simulink model "lego_code"  (R2018a)
settings: Solver=FixedStepDiscrete  StartTime=0.0  StopTime=Tsim  FixedStep=Ts  RelTol=1e-3
InitFcn:
  | singleinvertedpendulum
values from neighbouring files (symbols this model uses):
  K2 = -K2    [singleinvertedpendulum.m]
  R = 0.021    [singleinvertedpendulum.m]
  Ts = 0.001    [singleinvertedpendulum.m]
  x0 = [0;0.1;0;0]    [singleinvertedpendulum.m]
undefined symbols (not defined in the file or in its folder): Ad, Bd, Cd, Dd, Discrete, Time
libraries: legoev3lib x5, ctrlSharedLib x1
settings Model: ExtModeTrigDuration=2  Creator=srivats  LastModifiedBy=srivats
settings SolverCC: PositivePriorityOrder=on
settings OptimizationCC: EnhancedBackFolding=on  PassReuseOutputArgsAs=Individual arguments  MaxStackSize=64  OptimizeBlockOrder=speed  DifferentSizesBufferReuse=on  OptimizationCustomize=off
settings DebuggingCC: ParameterTunabilityLossMsg=error
settings HardwareCC: ProdBitPerPointer=32  ProdBitPerSizeT=32  ProdBitPerPtrDiffT=32  ProdLargestAtomicInteger=Long  ProdWordSize=32  ProdHWDeviceType=ARM Compatible->ARM 9
settings SFSimCC: MATLABDynamicMemAlloc=off
settings RTWCC: SystemTargetFile=ert.tlc  HardwareBoard=LEGO MINDSTORMS EV3  TLCOptions="-aInlineSetEventsForThisBaseRateFcn=TLC_FALSE -aSuppressMultiTaskScheduler=TLC_FALSE  -aRateBasedStepFcn=0"  TemplateMakefile=ert_default_tmf  GenerateReport=on  Toolchain=Sourcery G++ Lite v2009q3  IncludeHyperlinkInReport=on  LaunchReport=on  GenerateTraceInfo=on  GenerateTraceReport=on  GenerateTraceReportSl=on  GenerateTraceReportSf=on  GenerateTraceReportEml=on
settings CodeAppCC: ForceParamTrailComments=on  IgnoreCustomStorageClasses=off  OperatorAnnotations=on  SimulinkDataObjDesc=on  SFDataObjDesc=on  InsertBlockDesc=on
settings ERTTargetCC: SupportContinuousTime=on  SupportVariableSizeSignals=on

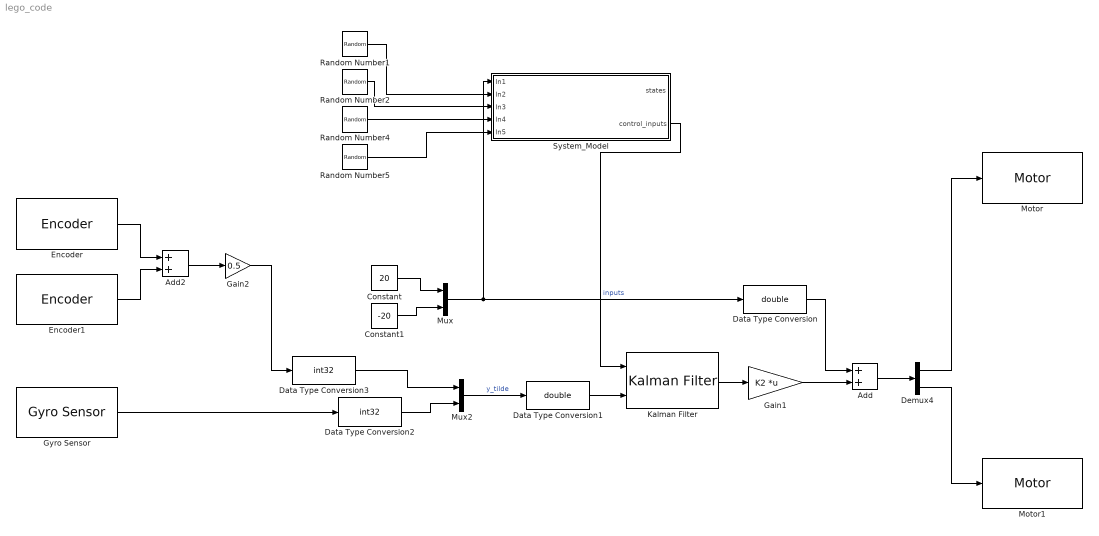
== system lego_code ==
  Add : Sum
  Add2 : Sum
  Constant : Constant  Value=20
  Constant1 : Constant  Value=-20
  Data Type Conversion : DataTypeConversion  OutDataTypeStr=double
  Data Type Conversion1 : DataTypeConversion  OutDataTypeStr=double
  Data Type Conversion2 : DataTypeConversion  OutDataTypeStr=int32
  Data Type Conversion3 : DataTypeConversion  OutDataTypeStr=int32
  Demux4 : Demux  Outputs=2
  Encoder : legoev3lib/Encoder  portNumber=A  opMode=Reset at each sample time  sampleTime=Ts
      settings: SourceProductName=Simulink Support Package for LEGO MINDSTORMS EV3 Hardware  SourceProductBaseCode=LEGOEV3
  Encoder1 : legoev3lib/Encoder  portNumber=D  opMode=Reset at each sample time  sampleTime=Ts
      settings: SourceProductName=Simulink Support Package for LEGO MINDSTORMS EV3 Hardware  SourceProductBaseCode=LEGOEV3
  Gain1 : Gain  Gain=K2  Multiplication=Matrix(K*u)
  Gain2 : Gain  Gain=0.5
  Gyro Sensor : legoev3lib/Gyro Sensor  portNumber=2  sampleTime=Ts
      settings: SourceProductName=Simulink Support Package for LEGO MINDSTORMS EV3 Hardware  SourceProductBaseCode=LEGOEV3
  Kalman Filter : ctrlSharedLib/Kalman Filter  TimeDomain=Discrete-Time  UseCurrentEstimator=on  ModelSource=Individual A, B, C, D matrices  ModelSourceVariable=ss(0.95,1,1,0,1)  A=Ad  B=Bd  C=Cd  D=Dd  NumberOfStates=4  NumberOfInputs=2  NumberOfOutputs=2  InitialEstimateSource=Dialog  X0=x0  P0=P0  UseK=off  UseGH=off  NumberOfProcessNoiseInputs=1  G=1  TimeInvariantG=on  H=0  TimeInvariantH=on  Q=Q  TimeInvariantQ=on  R=R  TimeInvariantR=on  N=0  TimeInvariantN=on  AddInputPort=on  AddEnablePort=off  OutputEstimatedY=off  OutputP=off  Ts=-1
      settings: SourceProductBaseCode=CT
  Motor : legoev3lib/Motor  sportNumber=A  sstopAction=Brake
  Motor1 : legoev3lib/Motor  sportNumber=D  sstopAction=Brake
  Mux : Mux  Inputs=2
  Mux2 : Mux  Inputs=2
  Random Number1 : RandomNumber  Variance=0.01  SampleTime=Ts
  Random Number2 : RandomNumber  Variance=0.025  Seed=1  SampleTime=Ts
  Random Number4 : RandomNumber  Variance=0.025  Seed=1  SampleTime=Ts
  Random Number5 : RandomNumber  Variance=0.025  Seed=1  SampleTime=Ts
  System_Model : Subsystem
  wires:
  Add/1 -> Demux4/1
  Kalman Filter/1 -> Gain1/1
  Demux4/1 -> Motor/1
  Gain1/1 -> Add/2
  Demux4/2 -> Motor1/1
  Data Type Conversion/1 -> Add/1
  Data Type Conversion1/1 -> Kalman Filter/2
  Constant1/1 -> Mux/2
  Constant/1 -> Mux/1
  Random Number2/1 -> System_Model/3(In3)
  Random Number5/1 -> System_Model/5(In5)
  Mux/1 -> System_Model/1(In1), Data Type Conversion/1  "inputs"
  Random Number1/1 -> System_Model/2(In2)
  Random Number4/1 -> System_Model/4(In4)
  System_Model/2(control_inputs) -> Kalman Filter/1
  Data Type Conversion3/1 -> Mux2/1
  Data Type Conversion2/1 -> Mux2/2
  Gain2/1 -> Data Type Conversion3/1
  Encoder1/1 -> Add2/2
  Gyro Sensor/1 -> Data Type Conversion2/1
  Mux2/1 -> Data Type Conversion1/1  "y_tilde"
  Add2/1 -> Gain2/1
  Encoder/1 -> Add2/1

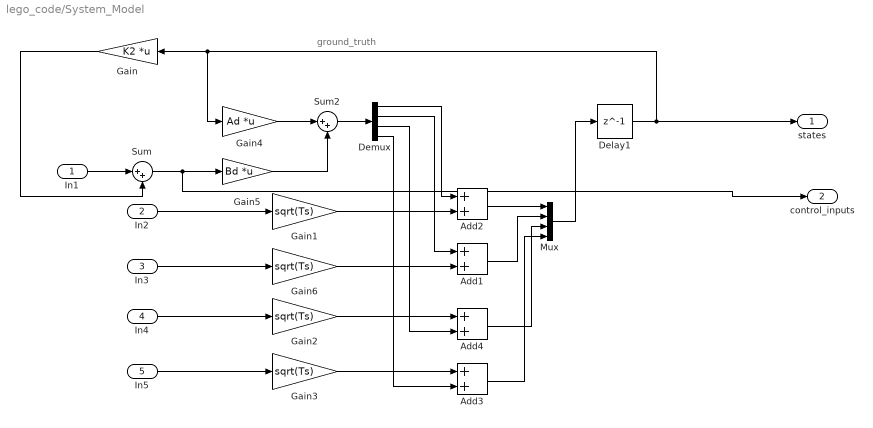
== system lego_code/System_Model ==
  note: ground_truth
  In1 : Inport
  In2 : Inport  Port=2
  In3 : Inport  Port=3
  In4 : Inport  Port=4
  In5 : Inport  Port=5
  Add{1..4} (4 alike) : Sum
  Delay1 : Delay  DelayLength=1  InitialCondition=x0  SampleTime=Ts
  Demux : Demux
  Gain : Gain  Gain=K2  Multiplication=Matrix(K*u)
  Gain{1..3,6} (4 alike) : Gain  Gain=sqrt(Ts)
  Gain4 : Gain  Gain=Ad  Multiplication=Matrix(K*u)
  Gain5 : Gain  Gain=Bd  Multiplication=Matrix(K*u)
  Mux : Mux
  Sum : Sum  Inputs=|++
  Sum2 : Sum  Inputs=|++
  states : Outport
  control_inputs : Outport  Port=2
  wires:
  Add1/1 -> Mux/2
  Gain4/1 -> Sum2/1
  Demux/2 -> Add1/1
  Gain1/1 -> Add2/2
  Sum2/1 -> Demux/1
  Add2/1 -> Mux/1
  Gain6/1 -> Add1/2
  In3/1 -> Gain6/1
  Mux/1 -> Delay1/1
  In2/1 -> Gain1/1
  Gain5/1 -> Sum2/2
  Demux/1 -> Add2/1
  In5/1 -> Gain3/1
  In4/1 -> Gain2/1
  Gain3/1 -> Add3/1
  Gain2/1 -> Add4/1
  Demux/3 -> Add4/2
  Demux/4 -> Add3/2
  Add4/1 -> Mux/3
  Add3/1 -> Mux/4
  In1/1 -> Sum/1
  Delay1/1 -> states/1, Gain/1, Gain4/1
  Gain/1 -> Sum/2
  Sum/1 -> control_inputs/1, Gain5/1
